simulink model "BasicTestModel"  (R2015a)
settings: Solver=ode3  StartTime=0.0  StopTime=10.0  FixedStep=1/200  RelTol=1e-3
undefined symbols (not defined in the file): i, Kd, Ki, Kp, Tf
libraries: PoliArd x8
settings Model: ExtModeTrigDuration=2  Creator=User  LastModifiedBy=user
settings OptimizationCC: OptimizeModelRefInitCode=on  LifeSpan=1
settings DebuggingCC: UnderspecifiedInitializationDetection=Classic  MergeDetectMultiDrivingBlocksExec=none
settings HardwareCC: ProdLargestAtomicInteger=Long  ProdLargestAtomicFloat=Double  ProdEndianess=LittleEndian  ProdHWDeviceType=ARM Compatible->ARM Cortex
settings RTWCC: SystemTargetFile=realtime.tlc  GenerateMakefile=off  TemplateMakefile=realtime.tmf  Description=Run on Target Hardware  RTWVerbose=off
settings ERTTargetCC: CombineOutputUpdateFcns=off  ExtModeTransport=3  ExtModeMexFile=ext_serial_win32_comm_rtt  ExtModeMexArgs=0 1 9600  ERTSrcFileBannerTemplate=realtime_code_template.cgt  ERTHdrFileBannerTemplate=realtime_code_template.cgt  ERTDataSrcFileTemplate=realtime_code_template.cgt  ERTDataHdrFileTemplate=realtime_code_template.cgt  ERTCustomFileTemplate=realtime_file_process.tlc

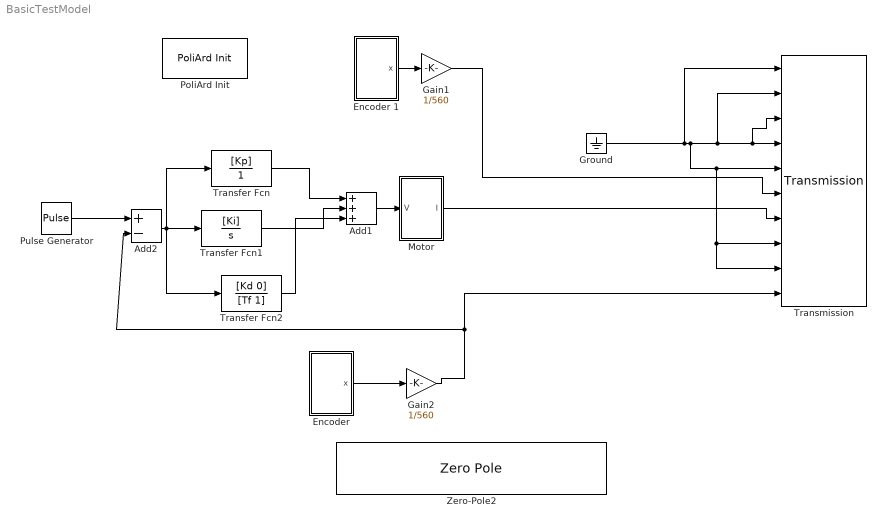
== system BasicTestModel ==
  Add1 : Sum  Inputs=+++
  Add2 : Sum  Inputs=+-
  "Encoder " : Subsystem
  Encoder 1 : Subsystem
  Gain1 : Gain  Gain=1/560
  Gain2 : Gain  Gain=1/560
  Ground : Ground
  Motor : Subsystem
  PoliArd Init : PoliArd/PoliArd Init
  Pulse Generator : DiscretePulseGenerator  PulseType=Time based  Period=10  PulseWidth=50
  Transfer Fcn : TransferFcn  Numerator=[Kp]  Denominator=1
  Transfer Fcn1 : TransferFcn  Numerator=[Ki]  Denominator=[1 0]
  Transfer Fcn2 : TransferFcn  Numerator=[Kd 0]  Denominator=[Tf 1]
  Transmission : PoliArd/Transmission  sample_freq=200  sig_to_send=6
  Zero-Pole2 : ZeroPole  Zeros=[-79.8,-33.1, -58.4+16.9*i , -58.4-16.9*i]  Poles=[0,-111,-566+45.7*i, -566-45.7*i]  Gain=-4.3815
  wires:
  Motor/1(I) -> Transmission/7
  "Encoder "/1(x) -> Gain2/1
  Gain2/1 -> Add2/2, Transmission/10
  Encoder 1/1(x) -> Gain1/1
  Gain1/1 -> Transmission/6
  Ground/1 -> Transmission/1, Transmission/8, Transmission/9, Transmission/5, Transmission/2, Transmission/3, Transmission/4
  Transfer Fcn2/1 -> Add1/3
  Transfer Fcn1/1 -> Add1/2
  Transfer Fcn/1 -> Add1/1
  Add2/1 -> Transfer Fcn1/1, Transfer Fcn2/1, Transfer Fcn/1
  Pulse Generator/1 -> Add2/1
  Add1/1 -> Motor/1(V)

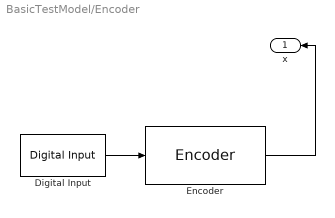
== system BasicTestModel/Encoder  ==
  Digital Input : PoliArd/Digital Input  DI_pin=2  DIsample=1/200
  Encoder : PoliArd/Encoder  EncoderID=4  dt_enc=-1
  x : Outport
  wires:
  Digital Input/1 -> Encoder/1
  Encoder/1 -> x/1

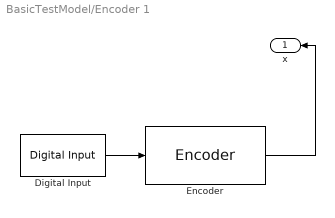
== system BasicTestModel/Encoder 1 ==
  Digital Input : PoliArd/Digital Input  DI_pin=2  DIsample=1/200
  Encoder : PoliArd/Encoder  EncoderID=3  dt_enc=-1
  x : Outport
  wires:
  Digital Input/1 -> Encoder/1
  Encoder/1 -> x/1

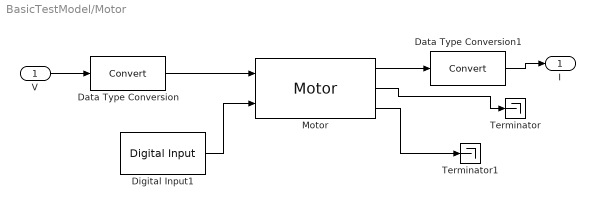
== system BasicTestModel/Motor ==
  V : Inport
  Data Type Conversion : DataTypeConversion
  Data Type Conversion1 : DataTypeConversion
  Digital Input1 : PoliArd/Digital Input  DI_pin=3  DIsample=1/200
  Motor : PoliArd/Motor  MotorID=2  DC_bus_mask=12  dt_mot=1/200
  Terminator : Terminator
  Terminator1 : Terminator
  I : Outport
  wires:
  Data Type Conversion/1 -> Motor/1
  Digital Input1/1 -> Motor/2
  V/1 -> Data Type Conversion/1
  Motor/3 -> Terminator1/1
  Motor/2 -> Terminator/1
  Motor/1 -> Data Type Conversion1/1
  Data Type Conversion1/1 -> I/1
